simulink model "HFI_UB_counter_latch"  (R2024a)
settings: Solver=FixedStepAuto  StartTime=0.0  StopTime=10  FixedStep=1e-6  RelTol=1e-3
values from neighbouring files (symbols this model uses):
  flux = 0.005753    [HFI_AVi.sldd]
  Ld = 0.00025    [HFI_AVi.sldd]
  Lq = 0.00056    [HFI_AVi.sldd]
  R = 0.6    [HFI_AVi.sldd]
undefined symbols (not defined in the file or in its folder): DiscIntNeverNeededParam, PI
libraries: simulink x3, slpidlib x3, powerlib_extras x2, spsDCVoltageSourceLib x1, spsGroundLib x1, spsPermanentMagnetSynchronousMachineLib x1, spsUniversalBridgeLib x1, sps_lib x1
(part 1 of 2)
settings Model: DataDictionary=HFI_AVi.sldd  Creator=Administrator  LastModifiedBy=cy
settings OptimizationCC: DefaultParameterBehavior=Inlined  UseDivisionForNetSlopeComputation=on  GainParamInheritBuiltInType=on  UseFloatMulNetSlope=on  InlineInvariantSignals=on  PassReuseOutputArgsAs=Individual arguments  ZeroExternalMemoryAtStartup=off  ZeroInternalMemoryAtStartup=off  NoFixptDivByZeroProtection=on  EfficientFloat2IntCast=on  LifeSpan=1  OptimizeBlockOrder=speed  DifferentSizesBufferReuse=on  EfficientTunableParamExpr=on
settings DebuggingCC: ParameterTunabilityLossMsg=error  UnconnectedInputMsg=warning  UnconnectedOutputMsg=warning  UnconnectedLineMsg=warning
settings HardwareCC: ProdBitPerPointer=32  ProdBitPerSizeT=32  ProdBitPerPtrDiffT=32  ProdLargestAtomicInteger=Long  ProdLargestAtomicFloat=Double  ProdWordSize=32  ProdLongLongMode=on  ProdHWDeviceType=ARM Compatible->ARM Cortex-M
settings ModelReferenceCC: EnableRefExpFcnMdlSchedulingChecks=on
settings SFSimCC: MATLABDynamicMemAlloc=off
settings RTWCC: Description=Embedded Coder  SystemTargetFile=ert.tlc  GenCodeOnly=on  TemplateMakefile=ert_default_tmf  GenerateReport=on  LaunchReport=on  GenerateCodeReplacementReport=on  GPUComputeCapability=3.5  DLArmComputeVersion=19.05
settings CodeAppCC: ForceParamTrailComments=on  IgnoreCustomStorageClasses=off  OperatorAnnotations=on  SimulinkDataObjDesc=on  SFDataObjDesc=on  CustomSymbolStrGlobalVar=rt$N$M  CustomSymbolStrType=$N$M  CustomSymbolStrFcn=$N$M$F  CustomSymbolStrMacro=$N$M  InsertBlockDesc=on
settings ERTTargetCC: TargetLangStandard=C99 (ISO)  CodeReplacementLibrary=ARM Cortex-M  GenerateSampleERTMain=on  IncludeMdlTerminateFcn=off  CombineSignalStateStructs=on  SupportComplex=off  SupportNonInlinedSFcns=on  InlinedParameterPlacement=NonHierarchical  ERTCustomFileTemplate=example_file_process.tlc  ERTFilePackagingFormat=CompactWithDataFile

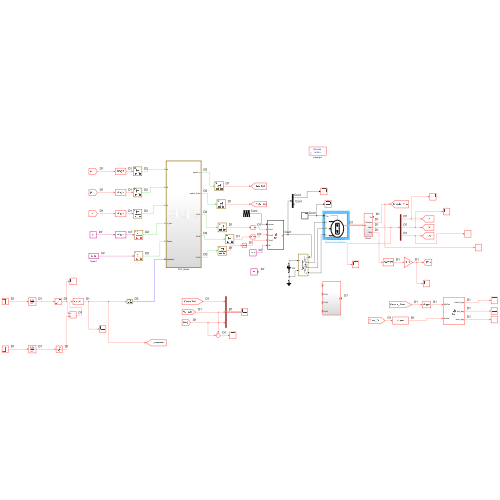
[thumbnail: Simulink's stored preview of the top-level diagram]
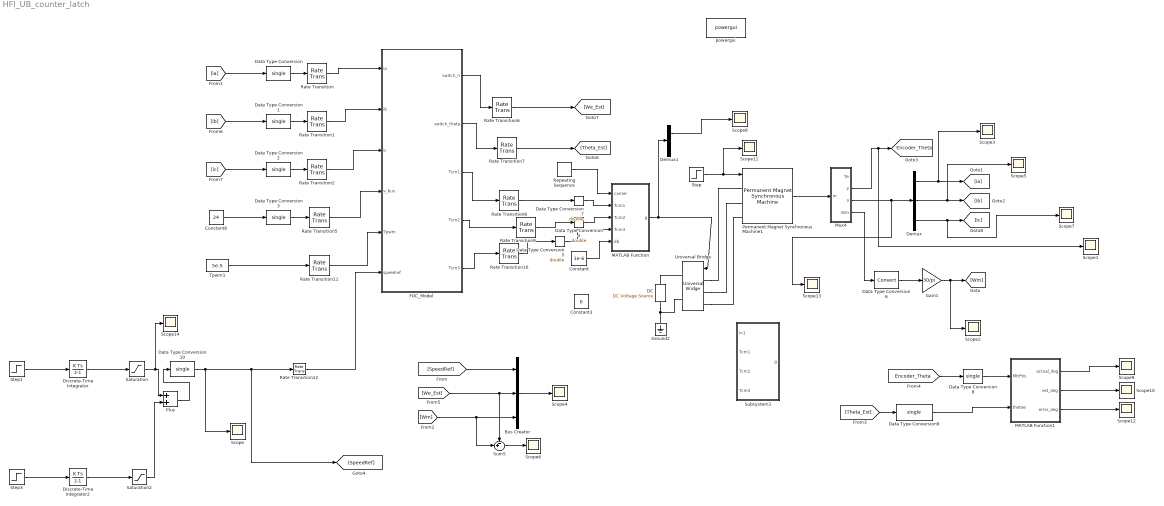
== system HFI_UB_counter_latch ==
  Bus Creator : BusCreator  Inputs=3
  Constant : Constant  Value=1e-6
  Constant3 : Constant  Value=0
  Constant6 : Constant  Value=24  OutDataTypeStr=single
  "DC " : spsDCVoltageSourceLib/DC Voltage Source  Amplitude=24  Measurements=None
  Data Type Conversion{,1..3,8..10} (7 alike) : DataTypeConversion  OutDataTypeStr=single  SaturateOnIntegerOverflow=off  RndMeth=Floor
  Data Type Conversion4 : DataTypeConversion  OutDataTypeStr=double  SaturateOnIntegerOverflow=off  RndMeth=Floor
  Data Type Conversion5 : DataTypeConversion  OutDataTypeStr=double  SaturateOnIntegerOverflow=off  RndMeth=Floor
  Data Type Conversion6 : DataTypeConversion  SaturateOnIntegerOverflow=off  RndMeth=Floor
  Data Type Conversion7 : DataTypeConversion  OutDataTypeStr=double  SaturateOnIntegerOverflow=off  RndMeth=Floor
  Demux : Demux  Outputs=3
  Demux1 : Demux  Outputs=[2 4]
  Discrete-Time Integrator : DiscreteIntegrator  SampleTime=-1  ICPrevOutput=DiscIntNeverNeededParam  ICPrevScaledInput=DiscIntNeverNeededParam
  Discrete-Time Integrator2 : DiscreteIntegrator  gainval=0.5  SampleTime=-1  ICPrevOutput=DiscIntNeverNeededParam  ICPrevScaledInput=DiscIntNeverNeededParam
  FOC_Model : Subsystem  TreatAsAtomicUnit=on
  Gain1 : Gain  Gain=30/pi
  Ground2 : spsGroundLib/Ground  LConnTagsString=a
  MATLAB Function : MATLAB Function  TreatAsAtomicUnit=on
  MATLAB Function1 : MATLAB Function  TreatAsAtomicUnit=on
  Mux4 : Subsystem
  Permanent Magnet Synchronous Machine1 : spsPermanentMagnetSynchronousMachineLib/Permanent Magnet Synchronous Machine  NbPhases=3  FluxDistribution=Sinusoidal  RotorType=Salient-pole  MechanicalLoad=Torque Tm  PresetModel=No  ShowDetailedParameters=on  MeasurementBus=off  Resistance=0.6  Inductance=0  dqInductances=[0.00025,0.00056]  La=[0.000279]  MachineConstant=Voltage Constant (V_peak L-L / krpm)  Flux=0.00572  VoltageCst=4.15  TorqueCst=0.03432  Flat=0  Mechanical=[4e-3,8e-4,4,1e-5]  PolePairs=4  InitialConditions=[0,0,0,0]  InitialConditions5ph=[0 0 0 0 0 0]  RefAngle=Aligned with phase A axis (original Park)  IterativeDiscreteModel=Trapezoidal non iterative  TsBlock=-1  TsPowergui=0
      link override From: GotoTag=T47_4340_3633560483959
      settings: AttributesFormatString=\n
  Plus : Sum
  Rate Transition{,1..2,5..12} (11 alike) : RateTransition
  Repeating Sequence : simulink/Sources/Repeating Sequence  rep_seq_t="[0  0.000025  0.00005]"  rep_seq_y="[0  0.000025  0]"
  Saturation : Saturate  UpperLimit=0  LowerLimit=-1000
  Saturation2 : Saturate  UpperLimit=2000  LowerLimit=0
  Scope{,1..14} (15 alike) : Scope
  Step : Step  Time=0  After=0  SampleTime=0
  Step1 : Step  Time=0.2  After=-1000
  Step3 : Step  Time=3  After=2000
  Subsystem1 : Subsystem
  Sum5 : Sum  Inputs=-+|
  Tpwm1 : Constant  Value=5e-5  OutDataTypeStr=single
  Universal Bridge : spsUniversalBridgeLib/Universal Bridge  Arms=3  SnubberResistance=1e5  SnubberCapacitance=inf  Device=IGBT / Diodes  Ron=1e-3  Lon=0  ForwardVoltages="[  0  0  ]"  ForwardVoltage=0  GTOparameters=[ 10e-6 , 20e-6 ]  IGBTparameters=[ 1e-6 , 2e-6 ]  Measurements=None  Measurements_2=None  converterType=Rectifier
  powergui : sps_lib/powergui  Priority=1  SimulationMode=Discrete  SampleTime=1e-6  frequency=60  Iterations=50  frequencyindice=0  Pbase=100e6  ErrMax=1e-4  UnitsV=kV  UnitsW=MW  buscounter=0  FunctionMessages=off  echomessages=off  EnableUseOfTLC=off  CurrentSourceSwitches=off  DisableSnubberDevices=off  DisableRonSwitches=off  DisableVfSwitches=off  DisplayEquations=off  AutomaticDiscreteSolvers=off  SolverType=Tustin/Backward Euler (TBE)  Interpol=off  ExternalGateDelay=off  methode=off  Ts=100  x0status=blocks  SPID=on  SwTol=0  HookPort=off  NonlinearTolerance=1e-4  nMaxIteration=100  ContinueOnMaxIteration=off  RestoreLinks=warning  ResistiveCurrentMeasurement=off  Frange=[0:2:500]  Ylog=off  Xlog=on  ShowGrid=off  save=off  variable=ZData  structure=0  ZoomFFT=off  StartTime=0.0  cycles=1  DisplayStyle=1  fundamental=60  FreqAxis=off  MaxFrequency=1000  frequencyindicesteady=1  RmsSteady=1  display=off
  tag scope: Encoder_Theta=global
  wires:
  [ia] -> Data Type Conversion/1
  [ic] -> Data Type Conversion2/1
  [ib] -> Data Type Conversion1/1
  Data Type Conversion/1 -> Rate Transition/1
  Data Type Conversion1/1 -> Rate Transition1/1
  Data Type Conversion2/1 -> Rate Transition2/1
  Constant6/1 -> Data Type Conversion3/1
  Rate Transition/1 -> FOC_Model/1(ia)
  Rate Transition1/1 -> FOC_Model/2(ib)
  Rate Transition2/1 -> FOC_Model/3(ic)
  Data Type Conversion3/1 -> Rate Transition5/1
  FOC_Model/2(switch_theta) -> Rate Transition7/1
  FOC_Model/1(switch_n) -> Rate Transition6/1
  Rate Transition5/1 -> FOC_Model/4(v_bus)
  Gain1/1 -> Scope2/1, [Wm]
  Data Type Conversion6/1 -> Gain1/1
  Data Type Conversion5/1 -> MATLAB Function/4(Tcm3)
  Data Type Conversion7/1 -> MATLAB Function/2(Tcm1)
  Mux4/4(Wm) -> Data Type Conversion6/1
  Demux/3 -> Scope7/1, [ic]
  Demux/2 -> Scope5/1, [ib]
  Mux4/3(Iabc) -> Scope13/1, Demux/1
  Demux/1 -> Scope3/1, [ia]
  Step/1 -> Scope11/1, Permanent Magnet Synchronous Machine1/1
  Permanent Magnet Synchronous Machine1/1 -> Mux4/1(m)
  Repeating Sequence/1 -> MATLAB Function/1(carrier)
  FOC_Model/3(Tcm1) -> Rate Transition8/1
  FOC_Model/4(Tcm2) -> Rate Transition9/1
  FOC_Model/5(Tcm3) -> Rate Transition10/1
  [We_Est] -> Sum5/1, Bus Creator/2
  [SpeedRef] -> Bus Creator/1
  [Wm] -> Sum5/2, Bus Creator/3
  Sum5/1 -> Scope6/1
  Bus Creator/1 -> Scope4/1
  Data Type Conversion8/1 -> MATLAB Function1/1(MtrPos)
  [Encoder_Theta] -> Data Type Conversion8/1
  [Theta_Est] -> Data Type Conversion9/1
  Mux4/2(Thetam) -> Scope1/1, [Encoder_Theta]
  Rate Transition6/1 -> [We_Est]
  Rate Transition7/1 -> [Theta_Est]
  Rate Transition8/1 -> Data Type Conversion7/1
  Rate Transition9/1 -> Data Type Conversion4/1
  Rate Transition10/1 -> Data Type Conversion5/1
  Tpwm1/1 -> Rate Transition11/1
  Rate Transition11/1 -> FOC_Model/5(Tpwm)
  Data Type Conversion9/1 -> MATLAB Function1/2(thetae)
  MATLAB Function/1(g) -> Universal Bridge/1, Demux1/1
  Data Type Conversion4/1 -> MATLAB Function/3(Tcm2)
  Demux1/1 -> Scope8/1
  Constant/1 -> MATLAB Function/5(db)
  MATLAB Function1/1(actual_deg) -> Scope9/1
  MATLAB Function1/2(est_deg) -> Scope10/1
  MATLAB Function1/3(error_deg) -> Scope12/1
  Discrete-Time Integrator2/1 -> Saturation2/1
  Plus/1 -> Data Type Conversion10/1
  Step3/1 -> Discrete-Time Integrator2/1
  Saturation2/1 -> Plus/2
  Discrete-Time Integrator/1 -> Saturation/1
  Data Type Conversion10/1 -> [SpeedRef], Rate Transition12/1, Scope/1
  Saturation/1 -> Scope14/1, Plus/1
  Step1/1 -> Discrete-Time Integrator/1
  Rate Transition12/1 -> FOC_Model/6(speedref)
  connections:
  "DC "/LConn1 -- Ground2/LConn1 -- Universal Bridge/RConn2
  Universal Bridge/LConn1 -- Permanent Magnet Synchronous Machine1/LConn1
  Universal Bridge/LConn3 -- Permanent Magnet Synchronous Machine1/LConn3
  Universal Bridge/LConn2 -- Permanent Magnet Synchronous Machine1/LConn2
  "DC "/RConn1 -- Universal Bridge/RConn1

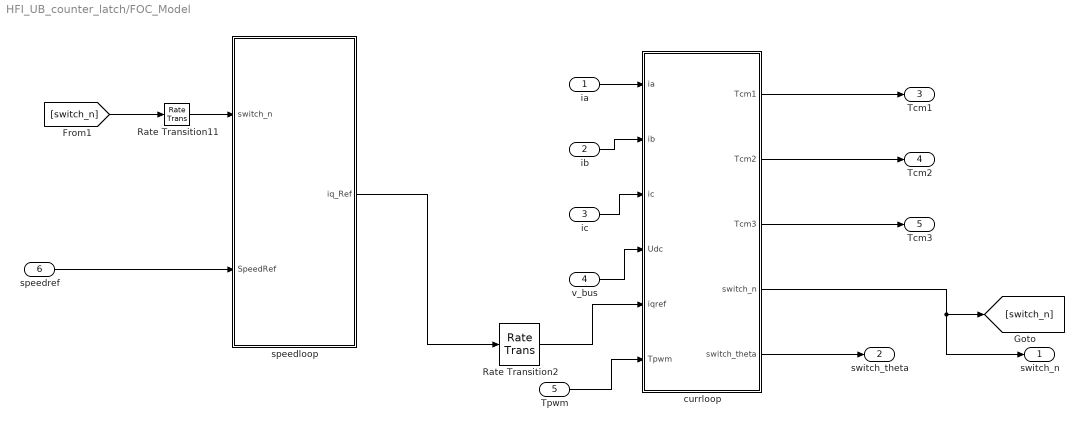
== system HFI_UB_counter_latch/FOC_Model ==
  ia : Inport
  ib : Inport  Port=2
  ic : Inport  Port=3
  v_bus : Inport  Port=4
  Tpwm : Inport  Port=5
  speedref : Inport  Port=6
  Rate Transition11 : RateTransition
  Rate Transition2 : RateTransition
  currloop : Subsystem  TreatAsAtomicUnit=on  SystemSampleTime=1e-4
  speedloop : Subsystem  TreatAsAtomicUnit=on  SystemSampleTime=1e-3
  switch_n : Outport
  switch_theta : Outport  Port=2
  Tcm1 : Outport  Port=3
  Tcm2 : Outport  Port=4
  Tcm3 : Outport  Port=5
  wires:
  ib/1 -> currloop/2(ib)
  ia/1 -> currloop/1(ia)
  Rate Transition2/1 -> currloop/5(iqref)
  ic/1 -> currloop/3(ic)
  v_bus/1 -> currloop/4(Udc)
  Rate Transition11/1 -> speedloop/1(switch_n)
  [switch_n] -> Rate Transition11/1
  speedref/1 -> speedloop/2(SpeedRef)
  speedloop/1(iq_Ref) -> Rate Transition2/1
  currloop/1(Tcm1) -> Tcm1/1
  currloop/2(Tcm2) -> Tcm2/1
  currloop/3(Tcm3) -> Tcm3/1
  Tpwm/1 -> currloop/6(Tpwm)
  currloop/4(switch_n) -> switch_n/1, [switch_n]
  currloop/5(switch_theta) -> switch_theta/1

== system HFI_UB_counter_latch/Mux4 ==
  m : Inport
  Bus Selector : BusSelector  OutputSignals=Stator current is_a (A),Stator current is_b (A),Stator current is_c (A)
  Bus Selector1 : BusSelector  OutputSignals=Rotor speed wm (rad/s),Rotor angle thetam (rad),Electromagnetic torque Te (N*m)
  Mux : Mux  Inputs=3
  Te : Outport
  Thetam : Outport  Port=2
  Iabc : Outport  Port=3
  Wm : Outport  Port=4
  wires:
  Mux/1 -> Iabc/1
  Bus Selector/1 -> Mux/1  "<Stator current is_a (A)>"
  Bus Selector/3 -> Mux/3  "<Stator current is_c (A)>"
  Bus Selector/2 -> Mux/2  "<Stator current is_b (A)>"
  m/1 -> Bus Selector1/1, Bus Selector/1
  Bus Selector1/3 -> Te/1  "<Electromagnetic torque Te (N*m)>"
  Bus Selector1/2 -> Thetam/1  "<Rotor angle thetam (rad)>"
  Bus Selector1/1 -> Wm/1  "<Rotor speed wm (rad/s)>"

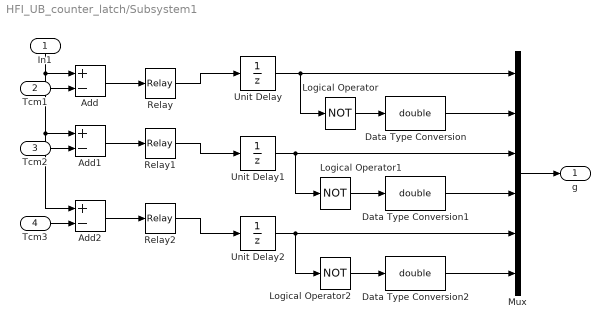
== system HFI_UB_counter_latch/Subsystem1 ==
  In1 : Inport
  Tcm1 : Inport  Port=2
  Tcm2 : Inport  Port=3
  Tcm3 : Inport  Port=4
  Add : Sum  Inputs=+-
  Add1 : Sum  Inputs=+-
  Add2 : Sum  Inputs=+-
  Data Type Conversion : DataTypeConversion  OutDataTypeStr=double  SaturateOnIntegerOverflow=off  RndMeth=Floor
  Data Type Conversion1 : DataTypeConversion  OutDataTypeStr=double  SaturateOnIntegerOverflow=off  RndMeth=Floor
  Data Type Conversion2 : DataTypeConversion  OutDataTypeStr=double  SaturateOnIntegerOverflow=off  RndMeth=Floor
  Logical Operator : Logic  Operator=NOT  AllPortsSameDT=off  OutDataTypeStr=boolean
  Logical Operator1 : Logic  Operator=NOT  AllPortsSameDT=off  OutDataTypeStr=boolean
  Logical Operator2 : Logic  Operator=NOT  AllPortsSameDT=off  OutDataTypeStr=boolean
  Mux : Mux  Inputs=6
  Relay : Relay  OffSwitchValue=-eps
  Relay1 : Relay  OffSwitchValue=-eps
  Relay2 : Relay  OffSwitchValue=-eps
  Unit Delay : UnitDelay  SampleTime=-1  HasFrameUpgradeWarning=on
  Unit Delay1 : UnitDelay  SampleTime=-1  HasFrameUpgradeWarning=on
  Unit Delay2 : UnitDelay  SampleTime=-1  HasFrameUpgradeWarning=on
  g : Outport  VectorParamsAs1DForOutWhenUnconnected=off
  wires:
  In1/1 -> Add1/1, Add2/1, Add/1
  Add/1 -> Relay/1
  Add2/1 -> Relay2/1
  Add1/1 -> Relay1/1
  Logical Operator/1 -> Data Type Conversion/1
  Logical Operator1/1 -> Data Type Conversion1/1
  Logical Operator2/1 -> Data Type Conversion2/1
  Data Type Conversion2/1 -> Mux/6
  Data Type Conversion1/1 -> Mux/4
  Data Type Conversion/1 -> Mux/2
  Mux/1 -> g/1
  Unit Delay/1 -> Mux/1, Logical Operator/1
  Unit Delay1/1 -> Logical Operator1/1, Mux/3
  Unit Delay2/1 -> Logical Operator2/1, Mux/5
  Relay/1 -> Unit Delay/1
  Relay1/1 -> Unit Delay1/1
  Relay2/1 -> Unit Delay2/1
  Tcm1/1 -> Add/2
  Tcm2/1 -> Add1/2
  Tcm3/1 -> Add2/2

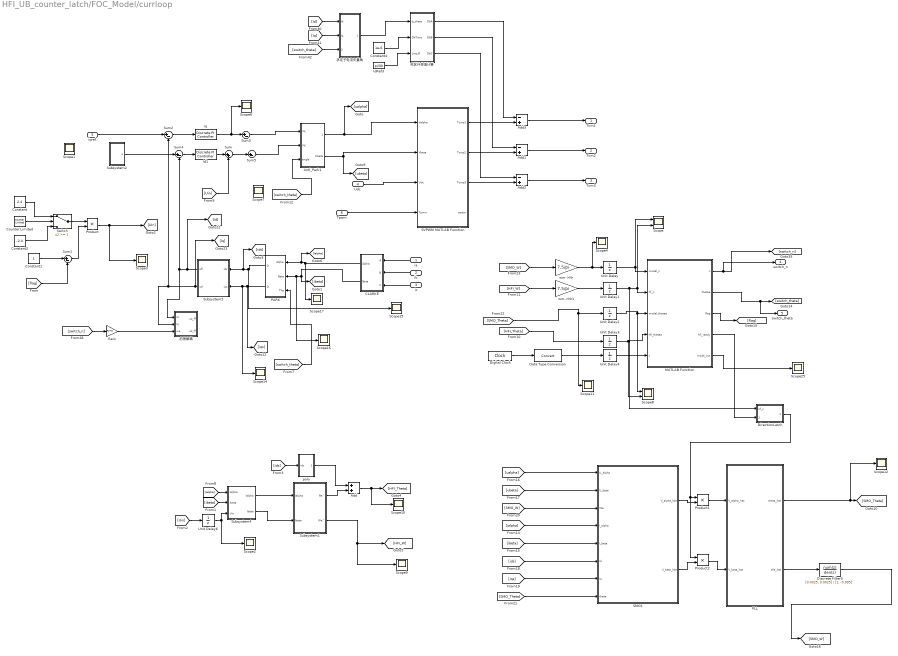
== system HFI_UB_counter_latch/FOC_Model/currloop ==
  ia : Inport
  ib : Inport  Port=2
  ic : Inport  Port=3
  Udc : Inport  Port=4
  iqref : Inport  Port=5
  Tpwm : Inport  Port=6
  Add : Sum
  Add1 : Sum  Inputs=-+
  Add2 : Sum  Inputs=-+
  Add3 : Sum  Inputs=-+
  Anti_Park1 : Subsystem
  CLARKE : Subsystem
  Constant : Constant  Value=2.4  OutDataTypeStr=single  SampleTime=-1
  Constant1 : Constant  OutDataTypeStr=single  SampleTime=-1
  Constant2 : Constant  Value=-2.4  OutDataTypeStr=single  SampleTime=-1
  Constant4 : Constant  Value=1e-6
  Counter Limited : simulink/Sources/Counter Limited  uplimit=1  tsamp=-1
  Data Type Conversion : DataTypeConversion  SaturateOnIntegerOverflow=off  RndMeth=Floor
  Digital Clock : DigitalClock  SampleTime=-1
  DirectionLatch : MATLAB Function  TreatAsAtomicUnit=on
  Discrete Filter5 : DiscreteFilter  Numerator=[0.0025, 0.0025]  Denominator=[1, -0.995]
  Gain : Gain  Gain=PI/7.5
  Id1 : powerlib_extras/Discrete  Control Blocks/Discrete PI Controller  Kp=0.00025*4000/2  Ki=0.6*4000/2  Par_Limits=[24*0.9*sqrt(1/3) -24*0.9*sqrt(1/3)]  Init=0  Ts=-1
  IdRef3 : Constant  Value=pi/30
  Iq : powerlib_extras/Discrete  Control Blocks/Discrete PI Controller  Kp=0.00056*4000/2  Ki=0.6*4000/2  Par_Limits=[24*0.9*sqrt(1/3) -24*0.9*sqrt(1/3)]  Init=0  Ts=-1
  MATLAB Function : MATLAB Function  TreatAsAtomicUnit=on
  PARK : Subsystem
  PLL : Subsystem
  Product : Product
  Product1 : Product  OutDataTypeStr=single
  Product2 : Product  OutDataTypeStr=single
  SMO1 : Subsystem
  SVPWM MATLAB Function : MATLAB Function  TreatAsAtomicUnit=on
  Scope : Scope  NumInputPorts=2
  Scope{1..4,6..7,9..12,14..17,25} (15 alike) : Scope
  Scope8 : Scope  NumInputPorts=2
  Subsystem1 : Subsystem
  Subsystem2 : Subsystem
  Subsystem4 : Subsystem
  Subsystem5 : Subsystem
  Sum : Sum  Inputs=|++
  Sum{1..5} (5 alike) : Sum  Inputs=|+-
  Switch : Switch  Threshold=1  SaturateOnIntegerOverflow=off  InputSameDT=off
  Unit Delay{,1..4,6} (6 alike) : UnitDelay  SampleTime=-1  HasFrameUpgradeWarning=on
  polo : Subsystem
  wm->Nr : Gain  Gain=7.5/pi
  wm->Nr1 : Gain  Gain=7.5/pi
  前馈解耦 : Subsystem
  死区补偿值计算 : Subsystem
  求定子电流矢量角 : Subsystem
  Tcm1 : Outport
  Tcm2 : Outport  Port=2
  Tcm3 : Outport  Port=3
  switch_n : Outport  Port=4
  switch_theta : Outport  Port=5
  wires:
  Anti_Park1/2(Ubeta) -> SVPWM MATLAB Function/2(Vbeta), [ubeta]
  CLARKE/1(Alpha) -> PARK/1(Alpha), [ialpha], Scope17/1
  Sum4/1 -> Id1/1
  Subsystem1/1(θe^) -> Add/2
  [switch_theta] -> PARK/3(The)
  ic/1 -> CLARKE/3(C)
  [ibeta] -> Subsystem4/2(ibeta)
  iqref/1 -> Sum2/1
  [ialpha] -> Subsystem4/1(ialpha)
  Subsystem1/2(We^) -> Scope9/1, [HFI_W]
  Sum2/1 -> Iq/1
  Subsystem4/1(Ialpha) -> Subsystem1/1(Ialpha)
  Anti_Park1/1(Ualpha) -> SVPWM MATLAB Function/1(Valpha), [ualpha]
  [Uin] -> Sum/2
  CLARKE/2(Beta) -> PARK/2(Beta), Scope16/1, [ibeta]
  ia/1 -> CLARKE/1(A)
  Subsystem4/2(Ibeta) -> Subsystem1/2(Ibeta)
  [switch_theta] -> Anti_Park1/3(angle)
  Add/1 -> Scope10/1, [HFI_Theta]
  Udc/1 -> SVPWM MATLAB Function/3(Udc)
  [ids] -> polo/1(ids)
  polo/1(Out1) -> Add/1
  ib/1 -> CLARKE/2(B)
  MATLAB Function/3(flag) -> [flag]
  [HFI_W] -> wm->Nr1/1
  Constant1/1 -> Sum1/1
  Constant/1 -> Switch/1
  Counter Limited/1 -> Switch/2
  Constant2/1 -> Switch/3
  Switch/1 -> Product/1
  [flag] -> Sum1/2
  Sum1/1 -> Product/2
  Digital Clock/1 -> Data Type Conversion/1
  MATLAB Function/1(n) -> switch_n/1, [switch_n]
  [ids] -> SMO1/6(Id)
  [iqs] -> SMO1/7(Iq)
  Iq/1 -> Sum3/1, Scope6/1
  Id1/1 -> Sum/1
  [ialpha] -> SMO1/4(I_alpha)
  [ibeta] -> SMO1/5(I_beta)
  Tpwm/1 -> SVPWM MATLAB Function/4(Tpwm)
  [Uin] -> Unit Delay6/1
  Subsystem2/1(id_Ref) -> Sum4/1
  [ualpha] -> SMO1/1(U_alpha)
  [ubeta] -> SMO1/2(U_beta)
  [SMO_W] -> SMO1/3(We)
  [SMO_Theta] -> SMO1/8(theta)
  PLL/1(theta_hat) -> Scope12/1, [SMO_Theta]
  PARK/1(D) -> Subsystem5/1(ids), [ids], Scope15/1
  PARK/2(Q) -> [iqs], Subsystem5/2(iqs), Scope14/1
  Subsystem5/1(idf) -> [Id], Sum4/2, 前馈解耦/1(id)
  Subsystem5/2(iqf) -> [Iq], 前馈解耦/2(iq), Sum2/2
  Gain/1 -> 前馈解耦/3(we)
  [switch_n] -> Gain/1
  Sum/1 -> Sum5/1
  Sum5/1 -> Anti_Park1/2(Vd)
  Sum3/1 -> Anti_Park1/1(Vq)
  wm->Nr/1 -> Scope4/1, Unit Delay/1
  Data Type Conversion/1 -> Unit Delay4/1
  Product/1 -> [Uin], Scope3/1
  Unit Delay6/1 -> Subsystem4/3(Uin), Scope2/1
  wm->Nr1/1 -> Unit Delay1/1
  Unit Delay/1 -> Scope/1, MATLAB Function/1(model_n)
  Unit Delay2/1 -> MATLAB Function/3(model_thetae), Scope8/1
  Unit Delay3/1 -> MATLAB Function/4(hfi_thetae), Scope8/2
  Unit Delay4/1 -> MATLAB Function/5(t)
  [HFI_Theta] -> Unit Delay3/1
  [SMO_W] -> wm->Nr/1
  [SMO_Theta] -> Scope11/1, Unit Delay2/1
  [Id] -> 求定子电流矢量角/1(Id)
  [Iq] -> 求定子电流矢量角/2(Iq)
  [switch_theta] -> 求定子电流矢量角/3(d_theta)
  求定子电流矢量角/1(theta) -> 死区补偿值计算/1(Is_theta)
  Constant4/1 -> 死区补偿值计算/2(DbTime)
  IdRef3/1 -> 死区补偿值计算/3(Line_θ)
  SVPWM MATLAB Function/3(Tcmp3) -> Add2/2
  Add2/1 -> Tcm3/1
  SVPWM MATLAB Function/2(Tcmp2) -> Add1/2
  Add1/1 -> Tcm2/1
  SVPWM MATLAB Function/1(Tcmp1) -> Add3/2
  Add3/1 -> Tcm1/1
  死区补偿值计算/1(DbA) -> Add3/1
  死区补偿值计算/2(DbB) -> Add1/1
  死区补偿值计算/3(DbC) -> Add2/1
  SMO1/2(V_beta_hat) -> Product2/2
  Product2/1 -> PLL/2(V_beta_hat)
  SMO1/1(V_alpha_hat) -> Product1/2
  Product1/1 -> PLL/1(V_alpha_hat)
  DirectionLatch/1(direction) -> Product2/1, Product1/1
  MATLAB Function/2(thetae) -> switch_theta/1, [switch_theta]
  MATLAB Function/4(hfi_ready) -> DirectionLatch/2(hfi_ready)
  MATLAB Function/5(mode_out) -> Scope25/1
  Unit Delay1/1 -> DirectionLatch/1(hf_n), Scope/2, MATLAB Function/2(hf_n)
  PLL/2(We_hat) -> Discrete Filter5/1
  Discrete Filter5/1 -> [SMO_W]

== system HFI_UB_counter_latch/FOC_Model/speedloop ==
  switch_n : Inport
  SpeedRef : Inport  Port=2
  Constant2 : Constant  Value=0
  Data Type Conversion : DataTypeConversion  OutDataTypeStr=single  SaturateOnIntegerOverflow=off  RndMeth=Floor
  Discrete PID Controller : slpidlib/PID Controller  Controller=PID  Form=Parallel  TimeDomain=Discrete-time  UseExternalTs=off  SampleTime=-1  IntegratorMethod=Forward Euler  FilterMethod=Forward Euler  ControllerParametersSource=internal  P=1  I=4  UseKiTs=off  D=0  UseExternalDerivativeSource=off  N=2  UseFilter=off  TunerSelectOption=Transfer Function Based (PID Tuner App)  InitialConditionSource=internal  InitialConditionForIntegrator=0  InitialConditionForFilter=0  DifferentiatorICPrevScaledInput=0  ExternalReset=none  TrackingMode=off  Kt=1  LimitOutput=on  SatLimitsSource=internal  UpperSaturationLimit=20  LowerSaturationLimit=-20  LinearizeAsGain=on  AntiWindupMode=back-calculation  Kb=1  LimitIntegrator=off  UpperIntegratorSaturationLimit=inf  LowerIntegratorSaturationLimit=-inf  POutMin=[]  POutMax=[]  IOutMin=[]  IOutMax=[]  DOutMin=[]  DOutMax=[]  NOutMin=[]  NOutMax=[]  SumOutMin=[]  SumOutMax=[]  SaturationOutMin=[]  SaturationOutMax=[]  PParamMin=[]  PParamMax=[]  IParamMin=[]  IParamMax=[]  DParamMin=[]  DParamMax=[]  NParamMin=[]  NParamMax=[]  KbParamMin=[]  KbParamMax=[]  KtParamMin=[]  KtParamMax=[]  KbOutMin=[]  KbOutMax=[]  KtOutMin=[]  KtOutMax=[]  IntegratorOutMin=[]  IntegratorOutMax=[]  FilterOutMin=[]  FilterOutMax=[]  SumI1OutMin=[]  SumI1OutMax=[]  SumI2OutMin=[]  SumI2OutMax=[]  SumI3OutMin=[]  SumI3OutMax=[]  SumI4OutMin=[]  SumI4OutMax=[]  SumDOutMin=[]  SumDOutMax=[]  DifferentiatorOutMin=[]  DifferentiatorOutMax=[]  FilterDiffOutCoefMin=[]  FilterDiffOutCoefMax=[]  ReciprocalOutMin=[]  ReciprocalOutMax=[]  SumDenOutMin=[]  SumDenOutMax=[]  SumNumOutMin=[]  SumNumOutMax=[]  DivideOutMin=[]  DivideOutMax=[]  UdiffTsProdOutMin=[]  UdiffTsProdOutMax=[]  NTsProdOutMin=[]  NTsProdOutMax=[]  UintegralTsProdOutMin=[]  UintegralTsProdOutMax=[]  UngainTsProdOutMin=[]  UngainTsProdOutMax=[]  ClampingZeroOutDataTypeStr=Inherit: Inherit via back propagation  ClampingZeroOutMin=[]  ClampingZeroOutMax=[]  FilterDenConstantOutDataTypeStr=Inherit: Inherit via back propagation  FilterDenConstantOutMin=[]  FilterDenConstantOutMax=[]  PCopyOutDataTypeStr=Inherit: Inherit via back propagation  PCopyOutMin=[]  PCopyOutMax=[]  NCopyOutDataTypeStr=Inherit: Inherit via back propagation  NCopyOutMin=[]  NCopyOutMax=[]  IntegratorContinuousStateAttributes=''  IntegratorStateMustResolveToSignalObject=off  IntegratorRTWStateStorageClass=Auto  FilterContinuousStateAttributes=''  FilterStateMustResolveToSignalObject=off  FilterRTWStateStorageClass=Auto  ParallelPVariant=InternalParameters  IdealPVariant=Disabled  IVariant=InternalParameters  DVariant=InternalParameters  IntegratorVariant=Discrete  SatVariant=Enabled  AWVariant=BackCalculation  PCopyVariant=Disabled  TRVariant=Disabled  FdbkBlocksVariant=Forward  IdealPFdbkVariant=Disabled  SatFdbkVariant=Disabled  DerivativeFilterVariant=Differentiator  NVariant=Passthrough  NCopyVariant=Disabled_SignalSpec  FilterICVariant=InternalICsDifferentiator  IntegratorICVariant=InternalICs  ExternalResetVariant=Disabled  TRSumVariant=Passthrough  SumFdbkVariant=Disabled  SumVariant=Sum_PID  TsampFilterVariant=InternalTs  TsampNgainVariant=Passthrough  TsampIntegralVariant=Disabled_SignalSpec  ExternalSaturationOutDataTypeStr=Inherit: Same as second input  DerivativeSourceVariant=ErrorSignal
      settings: LibrarySourceBlock=simulink/Discrete/Discrete PID Controller
  Mux1 : Mux  Inputs=2
  Scope2 : Scope
  Step2 : Step  Time=0.2  OutDataTypeStr=single
  Sum3 : Sum  Inputs=|+-
  Switch : Switch  Criteria=u2 > Threshold  SaturateOnIntegerOverflow=off  InputSameDT=off
  iq_Ref : Outport
  wires:
  SpeedRef/1 -> Mux1/1, Sum3/1
  Constant2/1 -> Data Type Conversion/1
  Data Type Conversion/1 -> Switch/3
  switch_n/1 -> Sum3/2, Mux1/2
  Sum3/1 -> Switch/1
  Discrete PID Controller/1 -> iq_Ref/1
  Step2/1 -> Switch/2
  Switch/1 -> Discrete PID Controller/1
  Mux1/1 -> Scope2/1

== system HFI_UB_counter_latch/FOC_Model/currloop/Anti_Park1 ==
  Vq : Inport
  Vd : Inport  Port=2
  angle : Inport  Port=3
  Fcn : Fcn  Expr=cos(u[1])*u[2]-sin(u[1])*u[3]
  Fcn1 : Fcn  Expr=sin(u[1])*u[2]+cos(u[1])*u[3]
  Mux1 : Mux  Inputs=3
  Ualpha : Outport
  Ubeta : Outport  Port=2
  wires:
  Fcn1/1 -> Ubeta/1
  Fcn/1 -> Ualpha/1
  Mux1/1 -> Fcn/1, Fcn1/1
  Vd/1 -> Mux1/2
  Vq/1 -> Mux1/3
  angle/1 -> Mux1/1

== system HFI_UB_counter_latch/FOC_Model/currloop/CLARKE ==
  A : Inport
  B : Inport  Port=2
  C : Inport  Port=3
  Mux : Mux  Inputs=3
  alpha : Fcn  Expr=(u(1)-0.5*(u(2)+u(3)))*2/3
  beta : Fcn  Expr=sqrt(3)/2*(u(2)-u(3))*2/3
  Alpha : Outport
  Beta : Outport  Port=2
  wires:
  alpha/1 -> Alpha/1
  B/1 -> Mux/2
  C/1 -> Mux/3
  A/1 -> Mux/1
  Mux/1 -> beta/1, alpha/1
  beta/1 -> Beta/1

== system HFI_UB_counter_latch/FOC_Model/currloop/PARK ==
  Alpha : Inport
  Beta : Inport  Port=2
  The : Inport  Port=3
  Mux : Mux  Inputs=3
  d : Fcn  Expr=u(1)*cos(u(3))+u(2)*sin(u(3))
  q : Fcn  Expr=-u(1)*sin(u(3))+u(2)*cos(u(3))
  D : Outport
  Q : Outport  Port=2
  wires:
  d/1 -> D/1
  Beta/1 -> Mux/2
  Alpha/1 -> Mux/1
  Mux/1 -> q/1, d/1
  q/1 -> Q/1
  The/1 -> Mux/3

== system HFI_UB_counter_latch/FOC_Model/currloop/PLL ==
  V_alpha_hat : Inport
  V_beta_hat : Inport  Port=2
  Add : Sum  Inputs=+-
  Discrete-Time Integrator : DiscreteIntegrator  SampleTime=-1  OutDataTypeStr=single  ICPrevOutput=DiscIntNeverNeededParam  ICPrevScaledInput=DiscIntNeverNeededParam
  Gain : Gain  Gain=-1
  PID Controller : slpidlib/PID Controller  Controller=PID  Form=Parallel  TimeDomain=Discrete-time  UseExternalTs=off  SampleTime=-1  IntegratorMethod=Forward Euler  FilterMethod=Forward Euler  ControllerParametersSource=internal  P=80  I=5000  UseKiTs=off  D=0  UseExternalDerivativeSource=off  N=0  UseFilter=on  TunerSelectOption=Transfer Function Based (PID Tuner App)  InitialConditionSource=internal  InitialConditionForIntegrator=0  InitialConditionForFilter=0  DifferentiatorICPrevScaledInput=0  ExternalReset=none  TrackingMode=off  Kt=1  LimitOutput=on  SatLimitsSource=internal  UpperSaturationLimit=1000  LowerSaturationLimit=-1000  LinearizeAsGain=on  AntiWindupMode=back-calculation  Kb=1  LimitIntegrator=off  UpperIntegratorSaturationLimit=inf  LowerIntegratorSaturationLimit=-inf  POutMin=[]  POutMax=[]  IOutMin=[]  IOutMax=[]  DOutMin=[]  DOutMax=[]  NOutMin=[]  NOutMax=[]  SumOutMin=[]  SumOutMax=[]  SaturationOutMin=[]  SaturationOutMax=[]  PParamMin=[]  PParamMax=[]  IParamMin=[]  IParamMax=[]  DParamMin=[]  DParamMax=[]  NParamMin=[]  NParamMax=[]  KbParamMin=[]  KbParamMax=[]  KtParamMin=[]  KtParamMax=[]  KbOutMin=[]  KbOutMax=[]  KtOutMin=[]  KtOutMax=[]  IntegratorOutMin=[]  IntegratorOutMax=[]  FilterOutMin=[]  FilterOutMax=[]  SumI1OutMin=[]  SumI1OutMax=[]  SumI2OutMin=[]  SumI2OutMax=[]  SumI3OutMin=[]  SumI3OutMax=[]  SumI4OutMin=[]  SumI4OutMax=[]  SumDOutMin=[]  SumDOutMax=[]  DifferentiatorOutMin=[]  DifferentiatorOutMax=[]  FilterDiffOutCoefMin=[]  FilterDiffOutCoefMax=[]  ReciprocalOutMin=[]  ReciprocalOutMax=[]  SumDenOutMin=[]  SumDenOutMax=[]  SumNumOutMin=[]  SumNumOutMax=[]  DivideOutMin=[]  DivideOutMax=[]  UdiffTsProdOutMin=[]  UdiffTsProdOutMax=[]  NTsProdOutMin=[]  NTsProdOutMax=[]  UintegralTsProdOutMin=[]  UintegralTsProdOutMax=[]  UngainTsProdOutMin=[]  UngainTsProdOutMax=[]  ClampingZeroOutDataTypeStr=Inherit: Inherit via back propagation  ClampingZeroOutMin=[]  ClampingZeroOutMax=[]  FilterDenConstantOutDataTypeStr=Inherit: Inherit via back propagation  FilterDenConstantOutMin=[]  FilterDenConstantOutMax=[]  PCopyOutDataTypeStr=Inherit: Inherit via back propagation  PCopyOutMin=[]  PCopyOutMax=[]  NCopyOutDataTypeStr=Inherit: Inherit via back propagation  NCopyOutMin=[]  NCopyOutMax=[]  IntegratorContinuousStateAttributes=''  IntegratorStateMustResolveToSignalObject=off  IntegratorRTWStateStorageClass=Auto  FilterContinuousStateAttributes=''  FilterStateMustResolveToSignalObject=off  FilterRTWStateStorageClass=Auto  ParallelPVariant=InternalParameters  IdealPVariant=Disabled  IVariant=InternalParameters  DVariant=InternalParameters  IntegratorVariant=Discrete  SatVariant=Enabled  AWVariant=BackCalculation  PCopyVariant=Disabled  TRVariant=Disabled  FdbkBlocksVariant=Forward  IdealPFdbkVariant=Disabled  SatFdbkVariant=Disabled  DerivativeFilterVariant=ForwardEulerFilter  NVariant=InternalParameters  NCopyVariant=Disabled  FilterICVariant=InternalICsFilter  IntegratorICVariant=InternalICs  ExternalResetVariant=Disabled  TRSumVariant=Passthrough  SumFdbkVariant=Disabled  SumVariant=Sum_PID  TsampFilterVariant=InternalTs  TsampNgainVariant=Passthrough  TsampIntegralVariant=Disabled_SignalSpec  ExternalSaturationOutDataTypeStr=Inherit: Same as second input  DerivativeSourceVariant=ErrorSignal
  Product : Product
  Product1 : Product
  Sin : Trigonometry
  Sin1 : Trigonometry  Operator=cos
  theta_hat : Outport
  We_hat : Outport  Port=2
  wires:
  Sin/1 -> Product1/2
  V_alpha_hat/1 -> Gain/1
  Product1/1 -> Add/2
  Sin1/1 -> Product/1
  V_beta_hat/1 -> Product1/1
  Product/1 -> Add/1
  Add/1 -> PID Controller/1
  Gain/1 -> Product/2
  Discrete-Time Integrator/1 -> theta_hat/1, Sin1/1, Sin/1
  PID Controller/1 -> Discrete-Time Integrator/1, We_hat/1

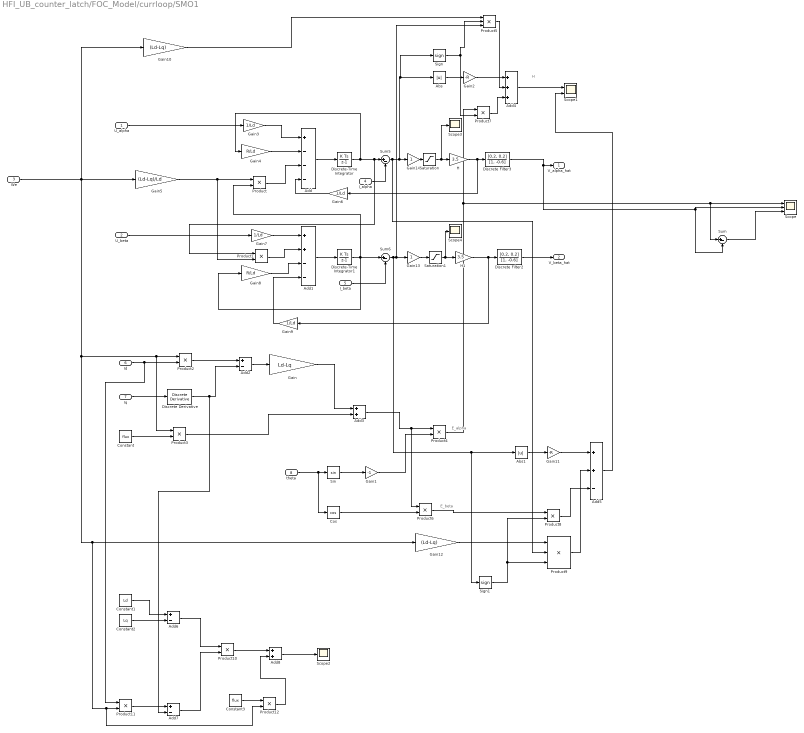
== system HFI_UB_counter_latch/FOC_Model/currloop/SMO1 ==
  note: H
  note: E_beta
  note: E_alpha
  U_alpha : Inport
  U_beta : Inport  Port=2
  We : Inport  Port=3
  I_alpha : Inport  Port=4
  I_beta : Inport  Port=5
  Id : Inport  Port=6
  Iq : Inport  Port=7
  theta : Inport  Port=8
  Abs : Abs  SaturateOnIntegerOverflow=off
  Abs1 : Abs  SaturateOnIntegerOverflow=off
  Add : Sum  Inputs=+---
  Add1 : Sum  Inputs=++--
  Add2 : Sum  Inputs=+-
  Add3 : Sum
  Add4 : Sum  Inputs=+++
  Add5 : Sum  Inputs=++-
  Add6 : Sum  Inputs=+-
  Add7 : Sum  Inputs=+-
  Add8 : Sum
  Constant : Constant  Value=flux  OutDataTypeStr=single
  Constant1 : Constant  Value=Ld  OutDataTypeStr=single
  Constant2 : Constant  Value=Lq  OutDataTypeStr=single
  Constant3 : Constant  Value=flux
  Cos : Trigonometry  Operator=cos
  Discrete Derivative : simulink/Discrete/Discrete Derivative  gainval=1.0  ICPrevScaledInput=0.0  OutMin=[]  OutMax=[]  OutDataType=fixdt(1, 16)  OutScaling=2^-10  DoSatur=off
  Discrete Filter2 : DiscreteFilter  Numerator=[0.2, 0.2]  Denominator=[1, -0.6]
  Discrete Filter3 : DiscreteFilter  Numerator=[0.2, 0.2]  Denominator=[1, -0.6]
  Discrete-Time Integrator : DiscreteIntegrator  SampleTime=-1  ICPrevOutput=DiscIntNeverNeededParam  ICPrevScaledInput=DiscIntNeverNeededParam
  Discrete-Time Integrator1 : DiscreteIntegrator  SampleTime=-1  ICPrevOutput=DiscIntNeverNeededParam  ICPrevScaledInput=DiscIntNeverNeededParam
  Gain : Gain  Gain=Ld-Lq
  Gain1 : Gain  Gain=-1
  Gain10 : Gain  Gain=(Ld-Lq)
  Gain11 : Gain  Gain=-R
  Gain12 : Gain  Gain=(Ld-Lq)
  Gain13 : Gain
  Gain14 : Gain
  Gain2 : Gain  Gain=-R
  Gain{3,6..7,9} (4 alike) : Gain  Gain=1/Ld
  Gain4 : Gain  Gain=R/Ld
  Gain5 : Gain  Gain=(Ld-Lq)/Ld
  Gain8 : Gain  Gain=R/Ld
  H : Gain  Gain=3.5
  H1 : Gain  Gain=3.5
  Product{,1..4,6..8,10..12} (11 alike) : Product
  Product5 : Product  Inputs=3
  Product9 : Product  Inputs=3
  Saturation : Saturate  UpperLimit=1  LowerLimit=-1
  Saturation1 : Saturate  UpperLimit=1  LowerLimit=-1
  Scope : Scope  NumInputPorts=3
  Scope1 : Scope  NumInputPorts=2
  Scope2 : Scope
  Scope3 : Scope
  Scope4 : Scope
  Sign : Signum
  Sign1 : Signum
  Sin : Trigonometry
  Sum : Sum  Inputs=|+-
  Sum5 : Sum  Inputs=|+-
  Sum6 : Sum  Inputs=|+-
  V_alpha_hat : Outport
  V_beta_hat : Outport  Port=2
  wires:
  U_beta/1 -> Gain7/1
  Gain8/1 -> Add1/3
  Gain5/1 -> Product/1, Product1/2
  Product1/1 -> Add1/2
  Discrete-Time Integrator1/1 -> Product/2, Sum6/1, Gain8/1
  Saturation1/1 -> Scope4/1, H1/1
  Product/1 -> Add/3
  Sum6/1 -> Abs1/1, Sign1/1, Gain13/1, Product5/3
  Discrete-Time Integrator/1 -> Product1/1, Sum5/1, Gain4/1
  Add/1 -> Discrete-Time Integrator/1
  Saturation/1 -> Scope3/1, H/1
  Gain3/1 -> Add/1
  Gain6/1 -> Add/4
  I_alpha/1 -> Sum5/2
  Gain4/1 -> Add/2
  Sum5/1 -> Product9/2, Sign/1, Abs/1, Gain14/1
  I_beta/1 -> Sum6/2
  U_alpha/1 -> Gain3/1
  Add1/1 -> Discrete-Time Integrator1/1
  Gain9/1 -> Add1/4
  Gain7/1 -> Add1/1
  Id/1 -> Product11/1, Product2/2
  Product2/1 -> Add2/1
  Iq/1 -> Discrete Derivative/1
  Discrete Derivative/1 -> Add7/2, Add2/2
  Add2/1 -> Gain/1
  Constant/1 -> Product3/2
  Product3/1 -> Add3/2
  Gain/1 -> Add3/1
  theta/1 -> Cos/1, Sin/1
  Sin/1 -> Gain1/1
  Add3/1 -> Product6/1, Product4/1
  Gain1/1 -> Product4/2
  Product4/1 -> Product7/1, Sum/1, Scope/1
  Cos/1 -> Product6/2
  Abs/1 -> Gain2/1
  Gain2/1 -> Add4/1
  Gain10/1 -> Product5/1
  Sign/1 -> Product5/2, Product7/2
  Product5/1 -> Add4/2
  Product7/1 -> Add4/3
  Add4/1 -> Scope1/1
  Abs1/1 -> Gain11/1
  Gain11/1 -> Add5/1
  Add5/1 -> Scope1/2
  Gain12/1 -> Product9/1
  Sign1/1 -> Product8/2, Product9/3
  Product9/1 -> Add5/2
  Product6/1 -> Product8/1
  Product8/1 -> Add5/3
  Constant1/1 -> Add6/1
  Constant2/1 -> Add6/2
  Add6/1 -> Product10/1
  Product11/1 -> Add7/1
  Add7/1 -> Product10/2
  Product10/1 -> Add8/1
  Constant3/1 -> Product12/1
  Product12/1 -> Add8/2
  Add8/1 -> Scope2/1
  Sum/1 -> Scope/3
  We/1 -> Product2/1, Product3/1, Product12/2, Product11/2, Gain12/1, Gain5/1, Gain10/1
  H1/1 -> Discrete Filter2/1, Gain9/1
  H/1 -> Discrete Filter3/1, Gain6/1
  Discrete Filter3/1 -> V_alpha_hat/1, Sum/2, Scope/2
  Discrete Filter2/1 -> V_beta_hat/1
  Gain13/1 -> Saturation1/1
  Gain14/1 -> Saturation/1

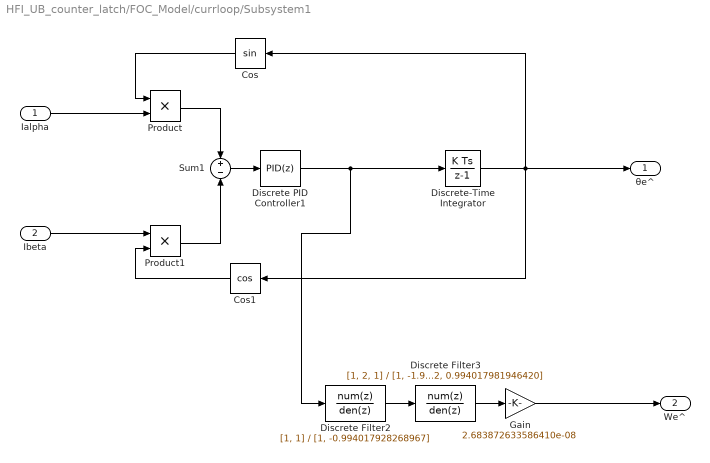
== system HFI_UB_counter_latch/FOC_Model/currloop/Subsystem1 ==
  Ialpha : Inport
  Ibeta : Inport  Port=2
  Cos : Trigonometry
  Cos1 : Trigonometry  Operator=cos
  Discrete Filter2 : DiscreteFilter  Numerator=[1, 1]  Denominator=[1, -0.994017928268967]
  Discrete Filter3 : DiscreteFilter  Numerator=[1, 2, 1]  Denominator=[1, -1.993982089730422, 0.994017981946420]
  Discrete PID Controller1 : slpidlib/PID Controller  Controller=PID  Form=Parallel  TimeDomain=Discrete-time  UseExternalTs=off  SampleTime=-1  IntegratorMethod=Forward Euler  FilterMethod=Forward Euler  ControllerParametersSource=internal  P=640  I=8600  UseKiTs=off  D=0  UseExternalDerivativeSource=off  N=100  UseFilter=off  TunerSelectOption=Transfer Function Based (PID Tuner App)  InitialConditionSource=internal  InitialConditionForIntegrator=0  InitialConditionForFilter=0  DifferentiatorICPrevScaledInput=0  ExternalReset=none  TrackingMode=off  Kt=1  LimitOutput=off  SatLimitsSource=internal  UpperSaturationLimit=inf  LowerSaturationLimit=-inf  LinearizeAsGain=off  AntiWindupMode=none  Kb=1  LimitIntegrator=off  UpperIntegratorSaturationLimit=inf  LowerIntegratorSaturationLimit=-inf  POutMin=[]  POutMax=[]  IOutMin=[]  IOutMax=[]  DOutMin=[]  DOutMax=[]  NOutMin=[]  NOutMax=[]  SumOutMin=[]  SumOutMax=[]  SaturationOutMin=[]  SaturationOutMax=[]  PParamMin=[]  PParamMax=[]  IParamMin=[]  IParamMax=[]  DParamMin=[]  DParamMax=[]  NParamMin=[]  NParamMax=[]  KbParamMin=[]  KbParamMax=[]  KtParamMin=[]  KtParamMax=[]  KbOutMin=[]  KbOutMax=[]  KtOutMin=[]  KtOutMax=[]  IntegratorOutMin=[]  IntegratorOutMax=[]  FilterOutMin=[]  FilterOutMax=[]  SumI1OutMin=[]  SumI1OutMax=[]  SumI2OutMin=[]  SumI2OutMax=[]  SumI3OutMin=[]  SumI3OutMax=[]  SumI4OutMin=[]  SumI4OutMax=[]  SumDOutMin=[]  SumDOutMax=[]  DifferentiatorOutMin=[]  DifferentiatorOutMax=[]  FilterDiffOutCoefMin=[]  FilterDiffOutCoefMax=[]  ReciprocalOutMin=[]  ReciprocalOutMax=[]  SumDenOutMin=[]  SumDenOutMax=[]  SumNumOutMin=[]  SumNumOutMax=[]  DivideOutMin=[]  DivideOutMax=[]  UdiffTsProdOutMin=[]  UdiffTsProdOutMax=[]  NTsProdOutMin=[]  NTsProdOutMax=[]  UintegralTsProdOutMin=[]  UintegralTsProdOutMax=[]  UngainTsProdOutMin=[]  UngainTsProdOutMax=[]  ClampingZeroOutDataTypeStr=Inherit: Inherit via back propagation  ClampingZeroOutMin=[]  ClampingZeroOutMax=[]  FilterDenConstantOutDataTypeStr=Inherit: Inherit via back propagation  FilterDenConstantOutMin=[]  FilterDenConstantOutMax=[]  PCopyOutDataTypeStr=Inherit: Inherit via back propagation  PCopyOutMin=[]  PCopyOutMax=[]  NCopyOutDataTypeStr=Inherit: Inherit via back propagation  NCopyOutMin=[]  NCopyOutMax=[]  IntegratorContinuousStateAttributes=''  IntegratorStateMustResolveToSignalObject=off  IntegratorRTWStateStorageClass=Auto  FilterContinuousStateAttributes=''  FilterStateMustResolveToSignalObject=off  FilterRTWStateStorageClass=Auto  ParallelPVariant=InternalParameters  IdealPVariant=Disabled  IVariant=InternalParameters  DVariant=InternalParameters  IntegratorVariant=Discrete  SatVariant=Disabled  AWVariant=Passthrough  PCopyVariant=Disabled  TRVariant=Disabled  FdbkBlocksVariant=Forward  IdealPFdbkVariant=Disabled  SatFdbkVariant=Disabled  DerivativeFilterVariant=Differentiator  NVariant=Passthrough  NCopyVariant=Disabled_SignalSpec  FilterICVariant=InternalICsDifferentiator  IntegratorICVariant=InternalICs  ExternalResetVariant=Disabled  TRSumVariant=Passthrough  SumFdbkVariant=Disabled  SumVariant=Sum_PID  TsampFilterVariant=InternalTs  TsampNgainVariant=Passthrough  TsampIntegralVariant=Disabled_SignalSpec  ExternalSaturationOutDataTypeStr=Inherit: Same as second input  DerivativeSourceVariant=ErrorSignal
      settings: LibrarySourceBlock=simulink/Discrete/Discrete PID Controller
  Discrete-Time Integrator : DiscreteIntegrator  SampleTime=-1  ICPrevOutput=DiscIntNeverNeededParam  ICPrevScaledInput=DiscIntNeverNeededParam
  Gain : Gain  Gain=2.683872633586410e-08
  Product : Product  OutDataTypeStr=single
  Product1 : Product  OutDataTypeStr=single
  Sum1 : Sum  Inputs=+|-  OutDataTypeStr=single  AccumDataTypeStr=single
  θe^ : Outport
  We^ : Outport  Port=2
  wires:
  Discrete Filter2/1 -> Discrete Filter3/1
  Discrete Filter3/1 -> Gain/1
  Discrete PID Controller1/1 -> Discrete-Time Integrator/1, Discrete Filter2/1
  Discrete-Time Integrator/1 -> Cos/1, Cos1/1, θe^/1
  Gain/1 -> We^/1
  Cos/1 -> Product/1
  Product/1 -> Sum1/1
  Ialpha/1 -> Product/2
  Ibeta/1 -> Product1/1
  Product1/1 -> Sum1/2
  Sum1/1 -> Discrete PID Controller1/1
  Cos1/1 -> Product1/2

== system HFI_UB_counter_latch/FOC_Model/currloop/Subsystem2 ==
  Add : Sum  Inputs=+-
  Add1 : Sum  Inputs=+-
  Add3 : Sum  Inputs=+-
  Step3 : Step  Time=0.1  After=2  OutDataTypeStr=single
  Step4 : Step  Time=0.11  After=2  OutDataTypeStr=single
  Step5 : Step  Time=0.13  After=2  OutDataTypeStr=single
  Step6 : Step  Time=0.14  After=2  OutDataTypeStr=single
  id_Ref : Outport
  wires:
  Step3/1 -> Add/1
  Step6/1 -> Add1/2
  Step4/1 -> Add/2
  Add/1 -> Add3/1
  Step5/1 -> Add1/1
  Add1/1 -> Add3/2
  Add3/1 -> id_Ref/1

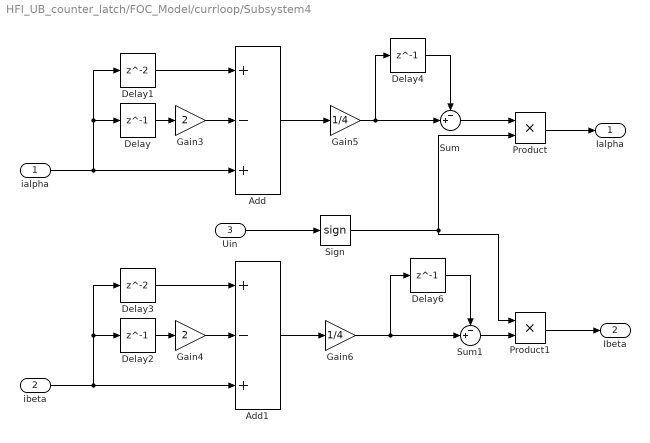
== system HFI_UB_counter_latch/FOC_Model/currloop/Subsystem4 ==
  ialpha : Inport
  ibeta : Inport  Port=2
  Uin : Inport  Port=3
  Add : Sum  Inputs=+-+
  Add1 : Sum  Inputs=+-+
  Delay{,2,4,6} (4 alike) : Delay  DelayLength=1  InitialCondition=0
  Delay1 : Delay  InitialCondition=0
  Delay3 : Delay  InitialCondition=0
  Gain3 : Gain  Gain=2
  Gain4 : Gain  Gain=2
  Gain5 : Gain  Gain=1/4
  Gain6 : Gain  Gain=1/4
  Product : Product  OutDataTypeStr=single
  Product1 : Product  OutDataTypeStr=single
  Sign : Signum
  Sum : Sum  Inputs=-+|
  Sum1 : Sum  Inputs=-+|
  Ialpha : Outport
  Ibeta : Outport  Port=2
  wires:
  Delay4/1 -> Sum/1
  Product/1 -> Ialpha/1
  Sum1/1 -> Product1/2
  Delay3/1 -> Add1/1
  Sum/1 -> Product/1
  Gain3/1 -> Add/2
  Uin/1 -> Sign/1
  Delay1/1 -> Add/1
  Add1/1 -> Gain6/1
  ibeta/1 -> Add1/3, Delay2/1, Delay3/1
  Add/1 -> Gain5/1
  Delay2/1 -> Gain4/1
  Gain4/1 -> Add1/2
  Gain6/1 -> Delay6/1, Sum1/2
  Delay6/1 -> Sum1/1
  Gain5/1 -> Sum/2, Delay4/1
  Delay/1 -> Gain3/1
  ialpha/1 -> Add/3, Delay/1, Delay1/1
  Sign/1 -> Product1/1, Product/2
  Product1/1 -> Ibeta/1

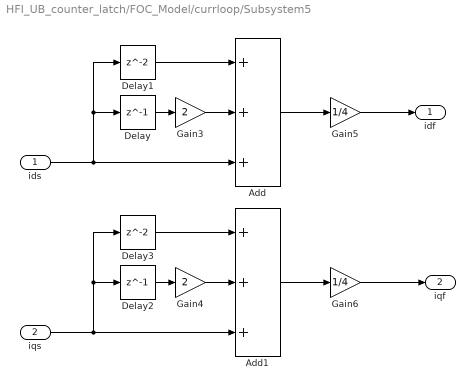
== system HFI_UB_counter_latch/FOC_Model/currloop/Subsystem5 ==
  ids : Inport
  iqs : Inport  Port=2
  Add : Sum  Inputs=+++
  Add1 : Sum  Inputs=+++
  Delay : Delay  DelayLength=1  InitialCondition=0
  Delay1 : Delay  InitialCondition=0
  Delay2 : Delay  DelayLength=1  InitialCondition=0
  Delay3 : Delay  InitialCondition=0
  Gain3 : Gain  Gain=2
  Gain4 : Gain  Gain=2
  Gain5 : Gain  Gain=1/4
  Gain6 : Gain  Gain=1/4
  idf : Outport
  iqf : Outport  Port=2
  wires:
  Delay2/1 -> Gain4/1
  Add1/1 -> Gain6/1
  Gain5/1 -> idf/1
  Delay1/1 -> Add/1
  iqs/1 -> Delay3/1, Delay2/1, Add1/3
  ids/1 -> Delay1/1, Delay/1, Add/3
  Gain6/1 -> iqf/1
  Add/1 -> Gain5/1
  Delay3/1 -> Add1/1
  Gain4/1 -> Add1/2
  Delay/1 -> Gain3/1
  Gain3/1 -> Add/2

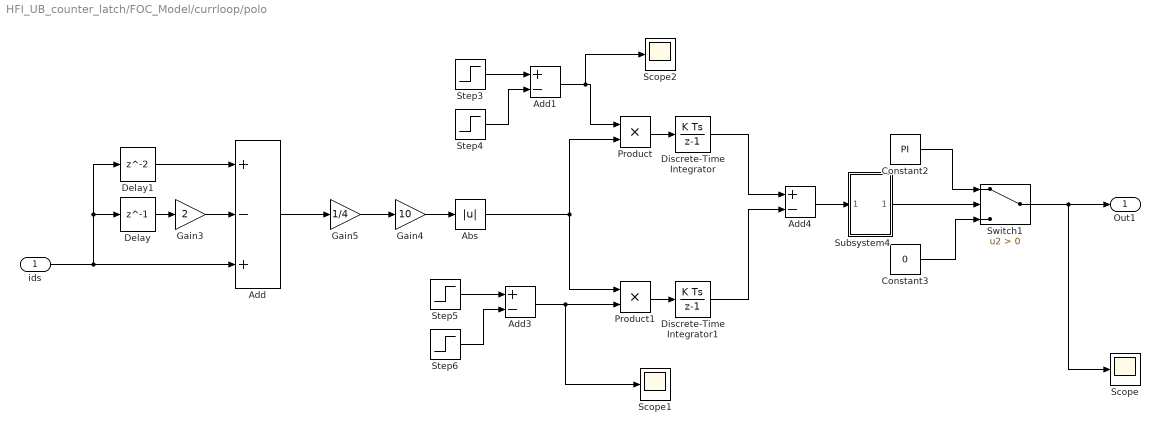
== system HFI_UB_counter_latch/FOC_Model/currloop/polo ==
  ids : Inport
  Abs : Abs  SaturateOnIntegerOverflow=off
  Add : Sum  Inputs=+-+
  Add1 : Sum  Inputs=+-
  Add3 : Sum  Inputs=+-
  Add4 : Sum  Inputs=+-
  Constant2 : Constant  Value=PI  OutDataTypeStr=single
  Constant3 : Constant  Value=0  OutDataTypeStr=single
  Delay : Delay  DelayLength=1  InitialCondition=0
  Delay1 : Delay  InitialCondition=0
  Discrete-Time Integrator : DiscreteIntegrator  SampleTime=-1  ICPrevOutput=DiscIntNeverNeededParam  ICPrevScaledInput=DiscIntNeverNeededParam
  Discrete-Time Integrator1 : DiscreteIntegrator  SampleTime=-1  ICPrevOutput=DiscIntNeverNeededParam  ICPrevScaledInput=DiscIntNeverNeededParam
  Gain3 : Gain  Gain=2
  Gain4 : Gain  Gain=10
  Gain5 : Gain  Gain=1/4
  Product : Product
  Product1 : Product
  Scope : Scope
  Scope1 : Scope
  Scope2 : Scope
  Step3 : Step  Time=0.1  OutDataTypeStr=single
  Step4 : Step  Time=0.11  OutDataTypeStr=single
  Step5 : Step  Time=0.13  OutDataTypeStr=single
  Step6 : Step  Time=0.14  OutDataTypeStr=single
  Subsystem4 : Subsystem
  Switch1 : Switch  Criteria=u2 > Threshold  SaturateOnIntegerOverflow=off  InputSameDT=off
  Out1 : Outport
  wires:
  Add4/1 -> Subsystem4/1(In1)
  Constant3/1 -> Switch1/3
  Step4/1 -> Add1/2
  Add3/1 -> Scope1/1, Product1/2
  Step5/1 -> Add3/1
  Discrete-Time Integrator1/1 -> Add4/2
  Step6/1 -> Add3/2
  Gain3/1 -> Add/2
  Add/1 -> Gain5/1
  Delay1/1 -> Add/1
  Delay/1 -> Gain3/1
  Gain5/1 -> Gain4/1
  ids/1 -> Add/3, Delay/1, Delay1/1
  Abs/1 -> Product/2, Product1/1
  Gain4/1 -> Abs/1
  Subsystem4/1(Out1) -> Switch1/2
  Product/1 -> Discrete-Time Integrator/1
  Step3/1 -> Add1/1
  Product1/1 -> Discrete-Time Integrator1/1
  Add1/1 -> Scope2/1, Product/1
  Discrete-Time Integrator/1 -> Add4/1
  Constant2/1 -> Switch1/1
  Switch1/1 -> Scope/1, Out1/1

== system HFI_UB_counter_latch/FOC_Model/currloop/前馈解耦 ==
  id : Inport
  iq : Inport  Port=2
  we : Inport  Port=3
  Gain : Gain  Gain=flux
  Gain1 : Gain  Gain=Ld
  Gain2 : Gain  Gain=Lq
  Product : Product
  Product1 : Product
  Sum : Sum  Inputs=|++
  uq_ff : Outport
  ud_ff : Outport  Port=2
  wires:
  Product1/1 -> ud_ff/1
  Gain2/1 -> Product1/1
  iq/1 -> Gain2/1
  Sum/1 -> uq_ff/1
  Gain/1 -> Sum/2
  Product/1 -> Sum/1
  id/1 -> Product/2
  Gain1/1 -> Product/1
  we/1 -> Gain1/1, Gain/1, Product1/2

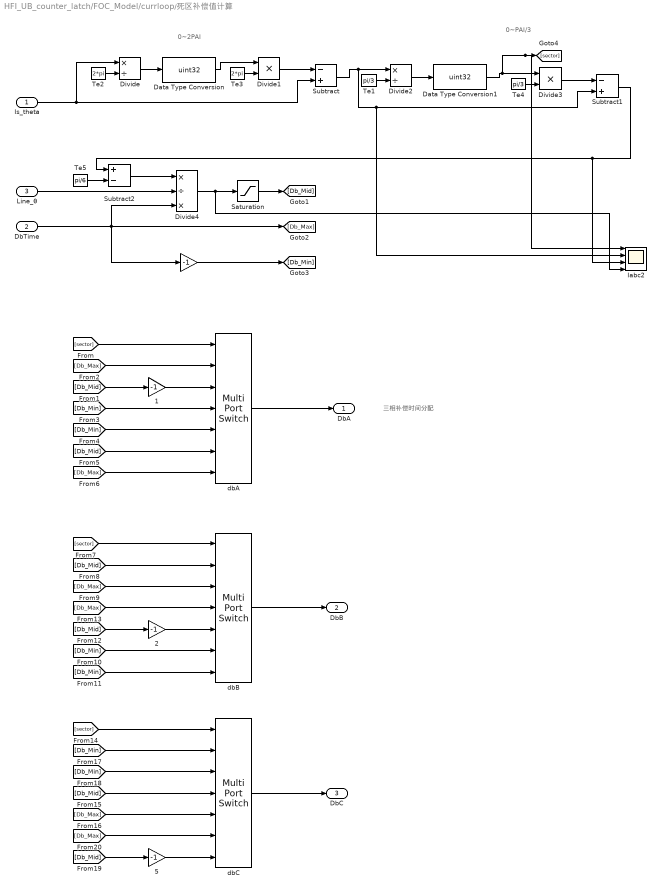
== system HFI_UB_counter_latch/FOC_Model/currloop/死区补偿值计算 ==
  note: 0~PAI/3
  note: 0~2PAI
  note: 三相补偿时间分配
  Is_theta : Inport
  DbTime : Inport  Port=2
  Line_θ : Inport  Port=3
   {,1..2,5} (4 alike) : Gain  Gain=-1
  Data Type Conversion : DataTypeConversion  OutDataTypeStr=uint32  SaturateOnIntegerOverflow=off  RndMeth=Floor
  Data Type Conversion1 : DataTypeConversion  OutDataTypeStr=uint32  SaturateOnIntegerOverflow=off  RndMeth=Floor
  Divide : Product  Inputs=*/
  Divide1 : Product  Inputs=**
  Divide2 : Product  Inputs=*/
  Divide3 : Product  Inputs=**
  Divide4 : Product  Inputs=*/*
  Iabc2 : Scope  NumInputPorts=4
  Saturation : Saturate  UpperLimit=0.8e-6  LowerLimit=-0.8e-6
  Subtract : Sum  Inputs=-+
  Subtract1 : Sum  Inputs=-+
  Subtract2 : Sum  Inputs=+-
  Te1 : Constant  Value=pi/3
  Te2 : Constant  Value=2*pi
  Te3 : Constant  Value=2*pi
  Te4 : Constant  Value=pi/3
  Te5 : Constant  Value=pi/6
  dbA : MultiPortSwitch  DataPortOrder=Zero-based contiguous  Inputs=6  zeroidx=on  SaturateOnIntegerOverflow=off  InputSameDT=off
  dbB : MultiPortSwitch  DataPortOrder=Zero-based contiguous  Inputs=6  zeroidx=on  SaturateOnIntegerOverflow=off  InputSameDT=off
  dbC : MultiPortSwitch  DataPortOrder=Zero-based contiguous  Inputs=6  zeroidx=on  SaturateOnIntegerOverflow=off  InputSameDT=off
  DbA : Outport
  DbB : Outport  Port=2
  DbC : Outport  Port=3
  wires:
  Saturation/1 -> [Db_Mid]
  " 2"/1 -> dbB/5
  [Db_Mid] -> dbB/2
  " 5"/1 -> dbC/7
  [Db_Min] -> dbB/6
  [Db_Min] -> dbA/4
  " 1"/1 -> dbA/3
  [Db_Mid] -> " 5"/1
  [Db_Max] -> dbC/6
  [Db_Max] -> dbC/5
  [Db_Mid] -> dbC/4
  [Db_Min] -> dbC/2
  [Db_Min] -> dbC/3
  [Db_Min] -> dbB/7
  [Db_Mid] -> " 2"/1
  [Db_Max] -> dbB/4
  [Db_Max] -> dbB/3
  dbA/1 -> DbA/1
  dbB/1 -> DbB/1
  dbC/1 -> DbC/1
  [sector] -> dbC/1
  [sector] -> dbB/1
  [Db_Max] -> dbA/7
  [Db_Mid] -> dbA/6
  [Db_Min] -> dbA/5
  [Db_Mid] -> " 1"/1
  [Db_Max] -> dbA/2
  [sector] -> dbA/1
  " "/1 -> [Db_Min]
  DbTime/1 -> Divide4/3, [Db_Max], " "/1
  Divide4/1 -> Saturation/1, Iabc2/4
  Line_θ/1 -> Divide4/2
  Subtract2/1 -> Divide4/1
  Subtract1/1 -> Subtract2/1, Iabc2/3
  Te5/1 -> Subtract2/2
  Divide3/1 -> Subtract1/1
  Data Type Conversion1/1 -> Divide3/1, Iabc2/1, [sector]
  Te4/1 -> Divide3/2
  Subtract/1 -> Divide2/1, Subtract1/2, Iabc2/2
  Divide2/1 -> Data Type Conversion1/1
  Te1/1 -> Divide2/2
  Te3/1 -> Divide1/2
  Divide/1 -> Data Type Conversion/1
  Te2/1 -> Divide/2
  Is_theta/1 -> Divide/1, Subtract/2
  Data Type Conversion/1 -> Divide1/1
  Divide1/1 -> Subtract/1

== system HFI_UB_counter_latch/FOC_Model/currloop/求定子电流矢量角 ==
  Id : Inport
  Iq : Inport  Port=2
  d_theta : Inport  Port=3
  Add : Sum
  Constant2 : Constant  Value=2*pi  OutDataTypeStr=single
  Id ~=0 : Subsystem
  Id= =0 : Subsystem
  If : If  IfExpression=u1 ~= 0
  If Action Subsystem : Subsystem  TreatAsAtomicUnit=on
  If Action Subsystem1 : Subsystem  TreatAsAtomicUnit=on
  Merge : Merge
  Mod1 : Math  Operator=mod  OutputSignalType=real
  theta : Outport
  wires:
  If Action Subsystem/1(Out1) -> Merge/2
  If Action Subsystem1/1(Out1) -> Merge/1
  Id ~=0/1(theta) -> If Action Subsystem1/1(In1)
  If/1 -> If Action Subsystem1/Action
  Id= =0/1(theta) -> If Action Subsystem/1(In1)
  Iq/1 -> Id= =0/1(iq), Id ~=0/1(iq)
  If/2 -> If Action Subsystem/Action
  Id/1 -> If/1, Id ~=0/2(id)
  Constant2/1 -> Mod1/2
  d_theta/1 -> Add/2
  Add/1 -> Mod1/1
  Mod1/1 -> theta/1
  Merge/1 -> Add/1

== system HFI_UB_counter_latch/FOC_Model/currloop/polo/Subsystem4 ==
  In1 : Inport
  CounterLatch150ms : MATLAB Function  TreatAsAtomicUnit=on
  Out1 : Outport
  wires:
  In1/1 -> CounterLatch150ms/1(u)
  CounterLatch150ms/1(y) -> Out1/1

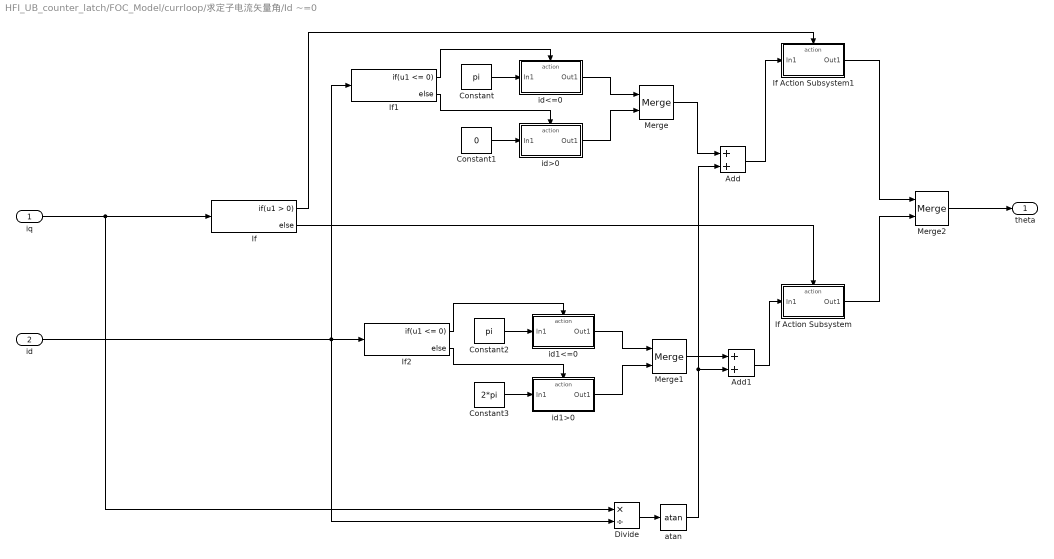
== system HFI_UB_counter_latch/FOC_Model/currloop/求定子电流矢量角/Id ~=0 ==
  iq : Inport
  id : Inport  Port=2
  Add : Sum  OutDataTypeStr=single  AccumDataTypeStr=single
  Add1 : Sum
  Constant : Constant  Value=pi  OutDataTypeStr=single
  Constant1 : Constant  Value=0  OutDataTypeStr=single
  Constant2 : Constant  Value=pi  OutDataTypeStr=single
  Constant3 : Constant  Value=2*pi  OutDataTypeStr=single
  Divide : Product  Inputs=*/
  If : If
  If Action Subsystem : Subsystem  TreatAsAtomicUnit=on
  If Action Subsystem1 : Subsystem  TreatAsAtomicUnit=on
  If1 : If  IfExpression=u1 <= 0
  If2 : If  IfExpression=u1 <= 0
  Merge : Merge
  Merge1 : Merge
  Merge2 : Merge
  atan : Trigonometry  Operator=atan
  id1<=0 : Subsystem  TreatAsAtomicUnit=on
  id1>0 : Subsystem  TreatAsAtomicUnit=on
  id<=0 : Subsystem  TreatAsAtomicUnit=on
  id>0 : Subsystem  TreatAsAtomicUnit=on
  theta : Outport
  wires:
  Add1/1 -> If Action Subsystem/1(In1)
  Merge1/1 -> Add1/1
  Add/1 -> If Action Subsystem1/1(In1)
  atan/1 -> Add/2, Add1/2
  Merge/1 -> Add/1
  Merge2/1 -> theta/1
  Divide/1 -> atan/1
  If Action Subsystem/1(Out1) -> Merge2/2
  If Action Subsystem1/1(Out1) -> Merge2/1
  Constant3/1 -> id1>0/1(In1)
  Constant2/1 -> id1<=0/1(In1)
  id1>0/1(Out1) -> Merge1/2
  id1<=0/1(Out1) -> Merge1/1
  If2/2 -> id1>0/Action
  If2/1 -> id1<=0/Action
  Constant1/1 -> id>0/1(In1)
  Constant/1 -> id<=0/1(In1)
  id>0/1(Out1) -> Merge/2
  id<=0/1(Out1) -> Merge/1
  If1/2 -> id>0/Action
  If1/1 -> id<=0/Action
  If/2 -> If Action Subsystem/Action
  If/1 -> If Action Subsystem1/Action
  id/1 -> If2/1, Divide/2, If1/1
  iq/1 -> Divide/1, If/1

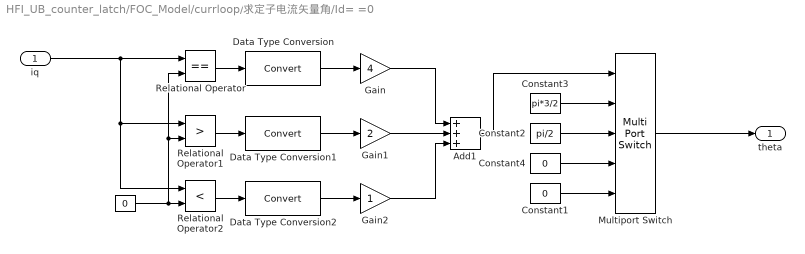
== system HFI_UB_counter_latch/FOC_Model/currloop/求定子电流矢量角/Id= =0 ==
  iq : Inport
  " " : Constant  Value=0  OutDataTypeStr=single
  Add1 : Sum  Inputs=+++
  Constant1 : Constant  Value=0  OutDataTypeStr=single
  Constant2 : Constant  Value=pi/2  OutDataTypeStr=single
  Constant3 : Constant  Value=pi*3/2  OutDataTypeStr=single
  Constant4 : Constant  Value=0  OutDataTypeStr=single
  Data Type Conversion : DataTypeConversion  SaturateOnIntegerOverflow=off  RndMeth=Floor
  Data Type Conversion1 : DataTypeConversion  SaturateOnIntegerOverflow=off  RndMeth=Floor
  Data Type Conversion2 : DataTypeConversion  SaturateOnIntegerOverflow=off  RndMeth=Floor
  Gain : Gain  Gain=4
  Gain1 : Gain  Gain=2
  Gain2 : Gain
  Multiport Switch : MultiPortSwitch  Inputs=4  SaturateOnIntegerOverflow=off  InputSameDT=off
  Relational Operator : RelationalOperator  Operator===  OutDataTypeStr=boolean  InputSameDT=off
  Relational Operator1 : RelationalOperator  Operator=>  OutDataTypeStr=boolean  InputSameDT=off
  Relational Operator2 : RelationalOperator  Operator=<  OutDataTypeStr=boolean  InputSameDT=off
  theta : Outport
  wires:
  Constant4/1 -> Multiport Switch/4
  Gain1/1 -> Add1/2
  Data Type Conversion2/1 -> Gain2/1
  Data Type Conversion1/1 -> Gain1/1
  Data Type Conversion/1 -> Gain/1
  Relational Operator2/1 -> Data Type Conversion2/1
  Relational Operator/1 -> Data Type Conversion/1
  Add1/1 -> Multiport Switch/1
  Gain2/1 -> Add1/3
  Gain/1 -> Add1/1
  Relational Operator1/1 -> Data Type Conversion1/1
  " "/1 -> Relational Operator2/2, Relational Operator1/2, Relational Operator/2
  iq/1 -> Relational Operator/1, Relational Operator1/1, Relational Operator2/1
  Constant3/1 -> Multiport Switch/2
  Constant2/1 -> Multiport Switch/3
  Constant1/1 -> Multiport Switch/5
  Multiport Switch/1 -> theta/1

== system HFI_UB_counter_latch/FOC_Model/currloop/求定子电流矢量角/If Action Subsystem ==
  In1 : Inport  OutDataTypeStr=single
  Action Port : ActionPort  ActionPortLabel=else
  Out1 : Outport
  wires:
  In1/1 -> Out1/1

== system HFI_UB_counter_latch/FOC_Model/currloop/求定子电流矢量角/If Action Subsystem1 ==
  In1 : Inport
  Action Port : ActionPort  ActionPortLabel=if(u1 ~= 0)
  Out1 : Outport  OutDataTypeStr=single
  wires:
  In1/1 -> Out1/1

== system HFI_UB_counter_latch/FOC_Model/currloop/求定子电流矢量角/Id ~=0/If Action Subsystem ==
  In1 : Inport
  Action Port : ActionPort  ActionPortLabel=else
  Out1 : Outport
  wires:
  In1/1 -> Out1/1

== system HFI_UB_counter_latch/FOC_Model/currloop/求定子电流矢量角/Id ~=0/If Action Subsystem1 ==
  In1 : Inport
  Action Port : ActionPort  ActionPortLabel=if(u1 > 0)
  Out1 : Outport
  wires:
  In1/1 -> Out1/1
